simulink subsystem "Control_Allocation"  (R2024b)
settings: Solver=VariableStepAuto  StartTime=0.0  StopTime=10.0  RelTol=1e-3
undefined symbols (not defined in the file): SimIn
libraries: simulink x1
settings Model: Creator=bmsimmon  LastModifiedBy=macheson
settings RTWCC: GPUComputeCapability=3.5

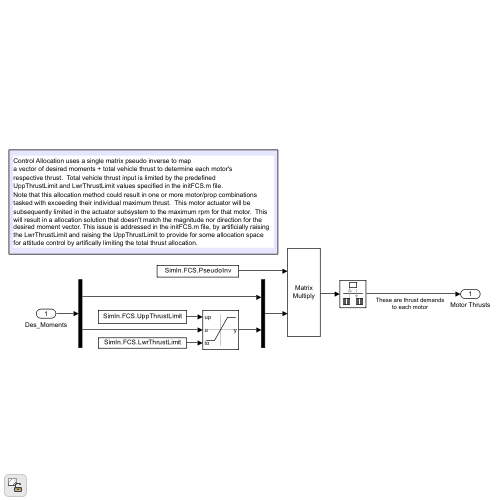
[thumbnail: Simulink's stored preview of the top-level diagram]
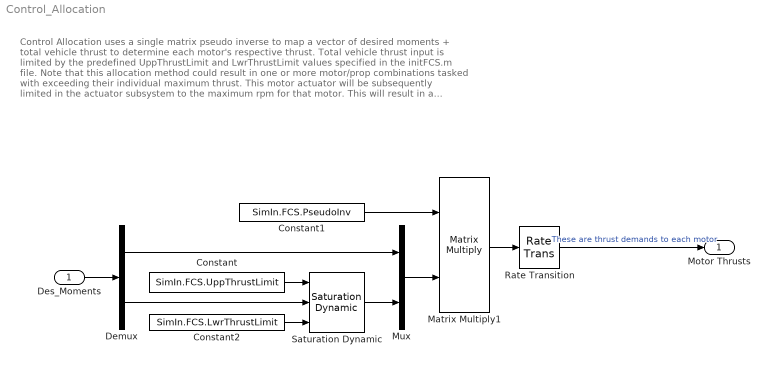
== system Control_Allocation ==
  note: Control Allocation uses a single matrix pseudo inverse to map
      | a vector of desired moments + total vehicle thrust to determine each motor's
      | respective thrust.  Total vehicle thrust input is limited by the predefined
      | UppThrustLimit and LwrThrustLimit values specified in the initFCS.m file.
      | Note that this allocation method could result in one or more motor/prop combinations
      | tasked with exceeding their individual maximum thrust.  This motor actuator will be
      | subsequently limited in the actuator subsystem to the maximum rpm for that motor.  This will result in a allocation solution that doesn't match the magnitude nor direction for the desired moment vector. This issue is addressed in the initFCS.m file, by artificially raising the LwrThrustLimit and raising the UppThrustLimit to provide for some allocation space for attitude control by artifically limiting the total thrust allocation.
  Des_Moments : Inport
  Constant : Constant  Value=SimIn.FCS.UppThrustLimit
  Constant1 : Constant  Value=SimIn.FCS.PseudoInv
  Constant2 : Constant  Value=SimIn.FCS.LwrThrustLimit
  Demux : Demux  Outputs=[3 1]
  Matrix Multiply1 : Product  Multiplication=Matrix(*)
  Mux : Mux  Inputs=2
  Rate Transition : RateTransition  OutPortSampleTime=SimIn.FCS.t_control
  Saturation Dynamic : simulink/Discontinuities/Saturation Dynamic  OutMin=[]  OutMax=[]  OutDataTypeStr=Inherit: Same as second input  OutDataType=fixdt(1, 16)  OutScaling=2^-10  DoSatur=off
  Motor Thrusts : Outport  VectorParamsAs1DForOutWhenUnconnected=off
  wires:
  Constant1/1 -> Matrix Multiply1/1
  Rate Transition/1 -> Motor Thrusts/1  "These are thrust demands to each motor"
  Matrix Multiply1/1 -> Rate Transition/1
  Des_Moments/1 -> Demux/1
  Demux/2 -> Saturation Dynamic/2
  Constant/1 -> Saturation Dynamic/1
  Saturation Dynamic/1 -> Mux/2
  Demux/1 -> Mux/1
  Mux/1 -> Matrix Multiply1/2
  Constant2/1 -> Saturation Dynamic/3
